simulink model "REPFF_test_sim"  (R2022b)
settings: Solver=FixedStepAuto  StartTime=0.0  StopTime=time_final  RelTol=1e-3
values from neighbouring files (symbols this model uses):
  controller_num = 2    [REPFF_test.m]
  Fzpet_den = F.Denominator{1}    [REPFF.m]
  Fzpet_num = F.Numerator{1}    [REPFF.m]
  K_aug = [K_SF,K_int]    [control_design.m]
  N1 = 2    [REPFF.m]
  signal_num = 2    [REPFF.m]    (also in REPFF_test.m)
  Stepsize = 0.4    [REPFF.m]    (also in REPFF_test.m; system_id_CLSOFCI.m)
  time_final = 20    [REPFF.m]    (also in REPFF_test.m; system_id_CLSOFCI.m)
  Ts = 0.001    [REPFF.m]    (also in REPFF_test.m; control_design.m; system_id_CLSOFCI.m)
  unit_period = 1    [REPFF.m]    (also in REPFF_test.m)
undefined symbols (not defined in the file or in its folder): A_d, Ad, B_d, Bd, C_d, L_Pred, N
libraries: simulink x1
settings Model: ExtModeTrigDuration=8  Creator=Alex Zhen  LastModifiedBy=Alex Zhen
settings OptimizationCC: DefaultUnderspecifiedDataType=single  EnhancedBackFolding=on  PassReuseOutputArgsAs=Individual arguments  MaxStackSize=1024  OptimizeBlockOrder=speed  DifferentSizesBufferReuse=on  OptimizationCustomize=off  DenormalBehavior=FlushToZero  EfficientTunableParamExpr=on
settings DebuggingCC: ParameterTunabilityLossMsg=error
settings HardwareCC: ProdBitPerChar=16  ProdBitPerInt=16  ProdBitPerPointer=32  ProdBitPerSizeT=32  ProdBitPerPtrDiffT=32  ProdLargestAtomicInteger=Integer  ProdLargestAtomicFloat=None  ProdWordSize=16  ProdLongLongMode=on  ProdHWDeviceType=Texas Instruments->C2000
settings SFSimCC: MATLABDynamicMemAlloc=off
settings RTWCC: Description=Embedded Coder  SystemTargetFile=ert.tlc  HardwareBoard=TI Delfino F28379D LaunchPad  TLCOptions=-aInlineSetEventsForThisBaseRateFcn=TLC_FALSE -aSuppressMultiTaskScheduler=TLC_FALSE -aRateBasedStepFcn=1  TemplateMakefile=ert_default_tmf  Toolchain=Texas Instruments Code Composer Studio (C2000)
settings CodeAppCC: ForceParamTrailComments=on  IgnoreCustomStorageClasses=off  OperatorAnnotations=on  SimulinkDataObjDesc=on  SFDataObjDesc=on  InsertBlockDesc=on
settings ERTTargetCC: CodeReplacementLibrary=TI C28x  SupportContinuousTime=on  ExtModeTransport=4  ExtModeStaticAlloc=on  ExtModeAutomaticAllocSize=off  ExtModeMexFile=ext_xcp  ExtModeIntrfLevel=Level2 - Open

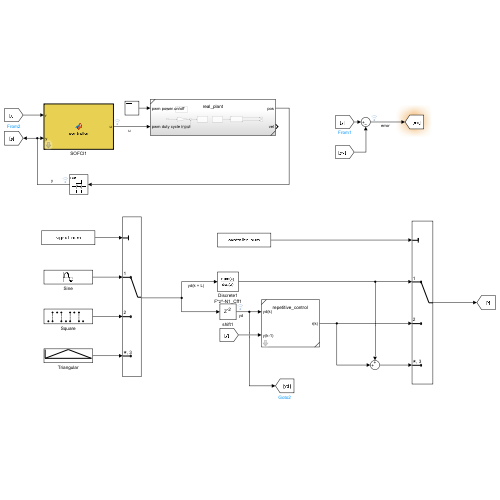
[thumbnail: Simulink's stored preview of the top-level diagram]
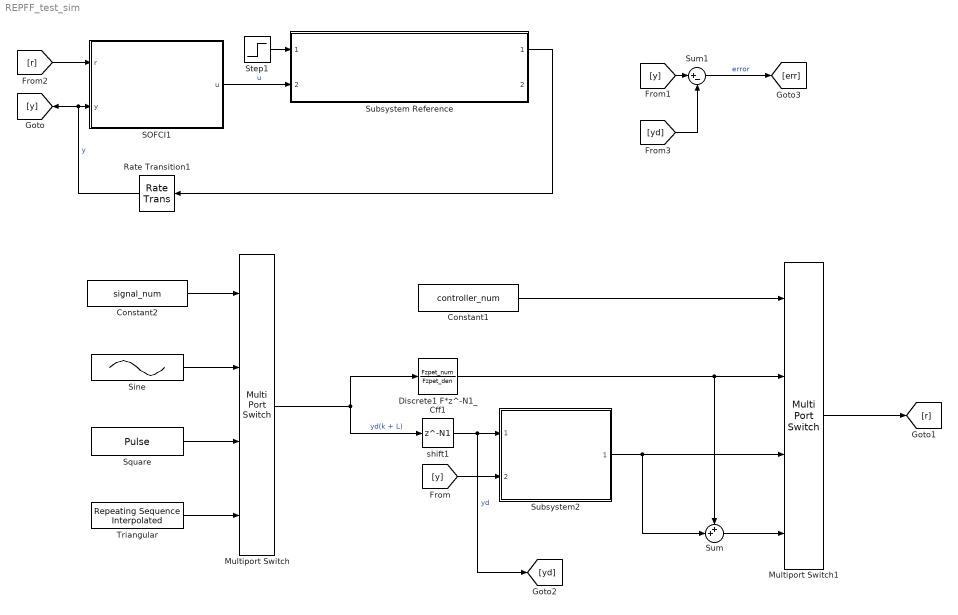
== system REPFF_test_sim ==
  Constant1 : Constant  Value=controller_num
  Constant2 : Constant  Value=signal_num
  Discrete1 F*z^-N1_Cff1 : DiscreteTransferFcn  Numerator=Fzpet_num  Denominator=Fzpet_den  SampleTime=Ts
  Multiport Switch : MultiPortSwitch  SaturateOnIntegerOverflow=off  InputSameDT=off
  Multiport Switch1 : MultiPortSwitch  SaturateOnIntegerOverflow=off  InputSameDT=off
  Rate Transition1 : RateTransition  Deterministic=off  OutPortSampleTime=Ts
  SOFCI1 : MATLAB Function  TreatAsAtomicUnit=on  mask{A=A_d, B=B_d, C=C_d, K=K_aug, L=L_Pred, N=N, Ad=Ad, Bd=Bd, linear_nonlinear=Nonlinear}
      mask prompts: linear_nonlinear "Linear/Nonlinear"
  Sine : Sin  Amplitude=Stepsize/2  Bias=Stepsize/2  Frequency=2*pi/(1/unit_period)  SampleTime=Ts
  Square : DiscretePulseGenerator  Amplitude=Stepsize  Period=1/Ts  PulseWidth=1/Ts/2  SampleTime=Ts
  Step1 : Step  Time=time_final  Before=1  After=0  SampleTime=0
  Subsystem Reference : Subsystem  ReferencedSubsystem=real_plant
  Subsystem2 : Subsystem  ReferencedSubsystem=repetitive_control  Np=Np  N1=N1  N2=N2  Fzpet_num=Fzpet_num  Fzpet_den=Fzpet_den  Q_coe=Q_coe  Qzpet_num=0  Qzpet_den=0
  Sum : Sum  Inputs=++|
  Sum1 : Sum  Inputs=|+-
  Triangular : simulink/Sources/Repeating Sequence Interpolated  OutValues=[0 Stepsize 0]  TimeValues=[0 unit_period/2 unit_period]  LookUpMeth=Interpolation-Use End Values  tsamp=Ts  OutMin=[]  OutMax=[]  OutDataTypeStr=double  OutputDataTypeScalingMode=double  OutDataType=fixdt(0,8)  OutScaling=2^-10
  shift1 : Delay  DelayLength=N1
  wires:
  [r] -> SOFCI1/1(r)
  Rate Transition1/1 -> [y], SOFCI1/2(y)  "y"
  Step1/1 -> Subsystem Reference/1
  SOFCI1/1(u) -> Subsystem Reference/2  "u"
  Subsystem Reference/1 -> Rate Transition1/1
  Sine/1 -> Multiport Switch/2
  Constant2/1 -> Multiport Switch/1
  Triangular/1 -> Multiport Switch/4
  Square/1 -> Multiport Switch/3
  Constant1/1 -> Multiport Switch1/1
  Subsystem2/1 -> Sum/2, Multiport Switch1/3
  Discrete1 F*z^-N1_Cff1/1 -> Multiport Switch1/2, Sum/1
  Multiport Switch1/1 -> [r]
  Multiport Switch/1 -> Discrete1 F*z^-N1_Cff1/1, shift1/1  "yd(k + L)"
  [y] -> Subsystem2/2
  Sum/1 -> Multiport Switch1/4
  shift1/1 -> [yd], Subsystem2/1  "yd"
  [yd] -> Sum1/2
  [y] -> Sum1/1
  Sum1/1 -> [err]  "error"

== matlab function REPFF_test_sim/SOFCI1 ==
  data: r input; u output; y input; A parameter; B parameter; C parameter; K parameter; L parameter; N parameter; Ad parameter; Bd parameter; linear_nonlinear parameter
function u = controller(r, y, A, B, C, K, L, N, Ad, Bd, linear_nonlinear)

persistent xhat xint;  %memory for the state

if isempty(xhat)  %local variable initialization
    n=size(L,1);
    xhat=zeros(n,1); 
    m = size(K,2) - n;
    xint=zeros(m,1);  
end

xaug=[xhat; xint]; %Augmented state include the state for the integrator

u_unsat = -K*xaug + N*r; %Control computation with integral action

if linear_nonlinear == 1
    u = u_unsat;
else
    u = sign(u_unsat)*min(1,abs(u_unsat));
end
%Update the next state next
xhat = (A-L*C)*xhat + B*u + L*y;
xint = Ad*xint + Bd*(y - r);
